simulink model "SIMControlleurMAT"  (Simulink 8.8)
settings: Solver=ode45  StartTime=0.0  StopTime=100  RelTol=1e-3  EnableMultiTasking=on
libraries: simulink x1
settings Model: Creator=Utilisateur-pc  LastModifiedBy=Jérôme
settings OptimizationCC: ExpressionDepthLimit=2147483647
settings DebuggingCC: SolverPrmCheckMsg=warning

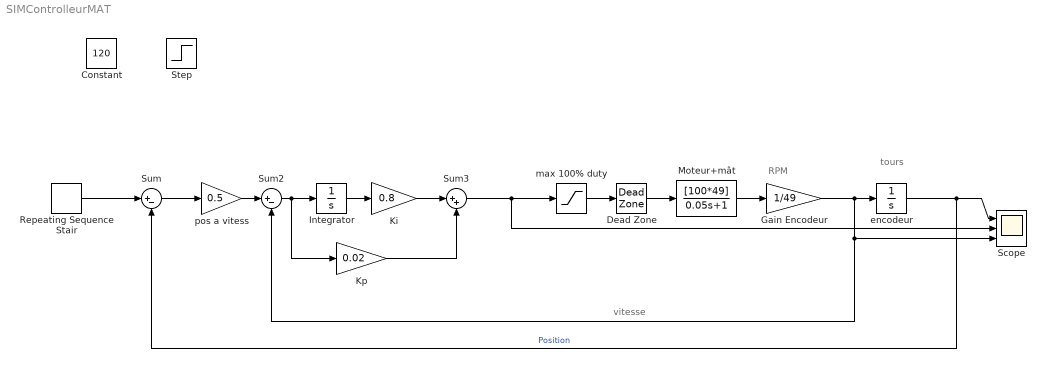
== system SIMControlleurMAT ==
  note: RPM
  note: tours
  note: vitesse
  Constant : Constant  Value=120  SampleTime=0.1
  "Dead Zone " : DeadZone  LowerValue=-0.1  UpperValue=0.1  SaturateOnIntegerOverflow=on
  Gain Encodeur : Gain  Gain=1/49
  Integrator : Integrator
  Ki : Gain  Gain=0.8
  Kp : Gain  Gain=0.02
  Moteur+mât : TransferFcn  Numerator=[100*49]  Denominator=[0.05 1]
  Repeating Sequence Stair : simulink/Sources/Repeating Sequence Stair  OutValues=[-170 170].'  tsamp=50  OutMin=[]  OutMax=[]  OutDataTypeStr=double  OutputDataTypeScalingMode=double  OutDataType=fixdt(0,8)  ConRadixGroup=Best Precision: Vector-wise  OutScaling=2^-12
  Scope : Scope  NumInputPorts=3
  Step : Step  Time=120  Before=-170  After=170  SampleTime=0.1  ZeroCross=off
  Sum : Sum  Inputs=|+-  SampleTime=0.1
  Sum2 : Sum  Inputs=|+-
  Sum3 : Sum  Inputs=|++
  encodeur : Integrator
  max 100% duty : Saturate  UpperLimit=1  LowerLimit=-1
  pos a vitess : Gain  Gain=0.5
  wires:
  Moteur+mât/1 -> Gain Encodeur/1
  encodeur/1 -> Scope/1, Sum/2  "Position"
  max 100% duty/1 -> "Dead Zone "/1
  "Dead Zone "/1 -> Moteur+mât/1
  pos a vitess/1 -> Sum2/1
  Sum2/1 -> Integrator/1, Kp/1
  Gain Encodeur/1 -> Scope/3, Sum2/2, encodeur/1
  Integrator/1 -> Ki/1
  Sum3/1 -> max 100% duty/1, Scope/2
  Kp/1 -> Sum3/2
  Sum/1 -> pos a vitess/1
  Ki/1 -> Sum3/1
  Repeating Sequence Stair/1 -> Sum/1
